simulink model "KENANLAB_20251017_184311"  (R2024a)
settings: Solver=VariableStepAuto  StartTime=0.0  StopTime=0.5  RelTol=1e-3
model workspace (MAT data in the model file):
  C2 = 23
undefined symbols (not defined in the file): K
settings Model: Creator=Sanan  LastModifiedBy=Sanan

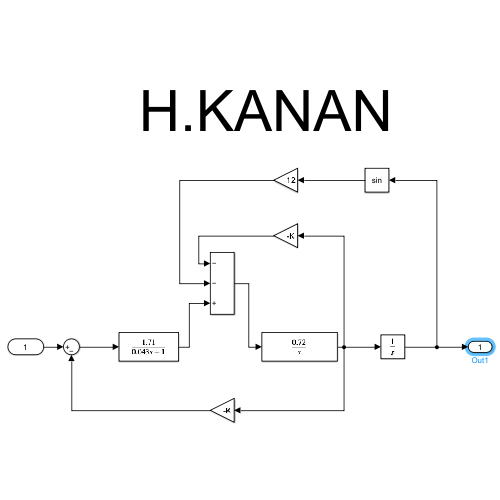
[thumbnail: Simulink's stored preview of the top-level diagram]
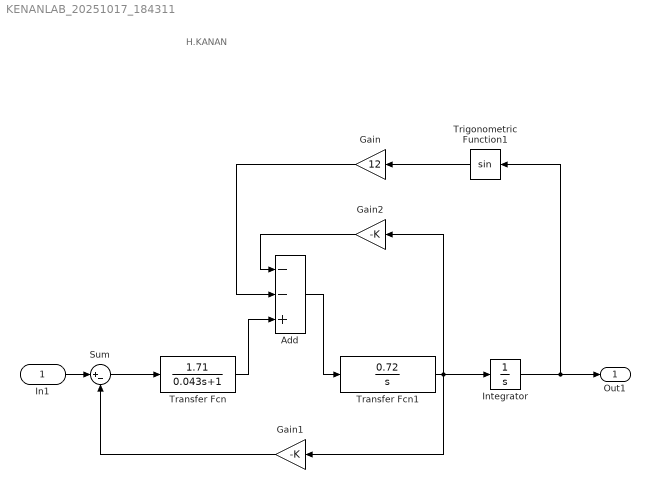
== system KENANLAB_20251017_184311 ==
  note: H.KANAN
  In1 : Inport
  Add : Sum  Inputs=--+
  Gain : Gain  Gain=12
  Gain1 : Gain  Gain=-K
  Gain2 : Gain  Gain=-K
  Integrator : Integrator
  Sum : Sum  Inputs=|+-
  Transfer Fcn : TransferFcn  Numerator=[1.71]  Denominator=[0.043 1]
  Transfer Fcn1 : TransferFcn  Numerator=[0.72]  Denominator=[1 0]
  Trigonometric Function1 : Trigonometry
  Out1 : Outport
  wires:
  In1/1 -> Sum/1
  Sum/1 -> Transfer Fcn/1
  Gain1/1 -> Sum/2
  Transfer Fcn1/1 -> Gain2/1, Gain1/1, Integrator/1
  Gain2/1 -> Add/1
  Gain/1 -> Add/2
  Transfer Fcn/1 -> Add/3
  Add/1 -> Transfer Fcn1/1
  Trigonometric Function1/1 -> Gain/1
  Integrator/1 -> Trigonometric Function1/1, Out1/1
